simulink model "DoorLockCntr"  (R2019b)
settings: Solver=FixedStepDiscrete  StartTime=0.0  StopTime=10.0  FixedStep=0.1  RelTol=1e-3  EnableMultiTasking=on
undefined symbols (not defined in the file or in its folder): LockStatus, SpeedCntVal, SpeedTh
libraries: simulink x5
settings Model: DataDictionary=DoorLockCntr.sldd  EnableAccessToBaseWorkspace=off  Creator=yyamamot  LastModifiedBy=tliang
settings DataIOCC: LimitDataPoints=on  SaveOutput=off  SaveTime=off  ReturnWorkspaceOutputs=off
settings OptimizationCC: DefaultParameterBehavior=Inlined  UseFloatMulNetSlope=on  UseSpecifiedMinMax=on  InlineInvariantSignals=on  PassReuseOutputArgsAs=Individual arguments  ZeroExternalMemoryAtStartup=off  ZeroInternalMemoryAtStartup=off  NoFixptDivByZeroProtection=on  EfficientFloat2IntCast=on  LifeSpan=1  EfficientTunableParamExpr=on
settings DebuggingCC: SFUnexpectedBacktrackingDiag=warning  SFNoUnconditionalDefaultTransitionDiag=warning  SFExecutionAtInitializationDiag=none  ArithmeticOperatorsInVariantConditions=warning
settings HardwareCC: ProdBitPerPointer=32  ProdBitPerSizeT=32  ProdBitPerPtrDiffT=32  ProdLargestAtomicFloat=None  ProdWordSize=32  ProdHWDeviceType=Generic->32-bit Embedded Processor
settings ModelReferenceCC: ModelReferenceNumInstancesAllowed=Single  PropagateSignalLabelsOutOfModel=off
settings SFSimCC: SimUseLocalCustomCode=off  MATLABDynamicMemAlloc=off  CustomCodeUndefinedFunction=UseInterfaceOnly
settings RTWCC: SystemTargetFile=ert.tlc  TemplateMakefile=ert_default_tmf  GenerateReport=on  RTWVerbose=off  RTWUseLocalCustomCode=off  BuildConfiguration=Faster Runs  IncludeHyperlinkInReport=on  LaunchReport=on  PortableWordSizes=on  GenerateTraceInfo=on  GenerateTraceReport=on  GenerateTraceReportSl=on  GenerateTraceReportSf=on  GenerateTraceReportEml=on  GenerateWebview=on  GenerateCodeMetricsReport=on
settings CodeAppCC: IgnoreCustomStorageClasses=off  StateflowObjectComments=on  ReqsInCode=on
settings ERTTargetCC: UtilityFuncGeneration=Shared location  MultiwordLength=2048  GenerateSampleERTMain=on  IncludeMdlTerminateFcn=off  CombineSignalStateStructs=on  SuppressErrorStatus=on  SupportAbsoluteTime=off  SupportNonFinite=off  SupportComplex=off  ERTCustomFileTemplate=example_file_process.tlc  ERTFilePackagingFormat=Compact
settings ConfigComp: CovScope=ReferencedModels  CovIncludeTopModel=off  CovMetricSettings=dw  CovHtmlReporting=on  CovSaveCumulativeToWorkspaceVar=on  CovSaveSingleToWorkspaceVar=on  CovExternalEMLEnable=off  DVModelCoverageObjectives=MCDC  DVMaxTestCaseSteps=500  DVTestSuiteOptimization=LongTestcases

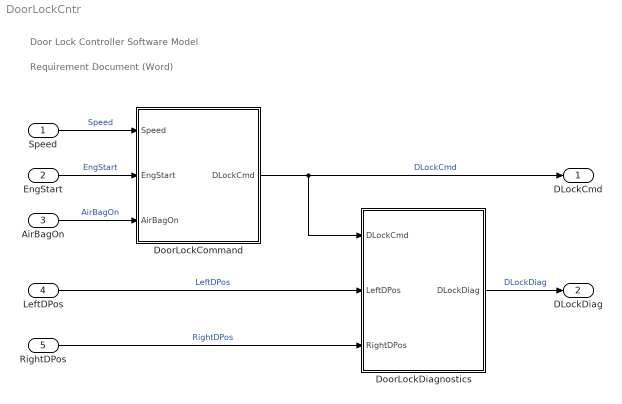
== system DoorLockCntr ==
  note: Door Lock Controller Software Model
  note: Requirement Document (Word)
  Speed : Inport  OutDataTypeStr=single  PortDimensions=1  SampleTime=0.1
  EngStart : Inport  Port=2  OutDataTypeStr=boolean  PortDimensions=1  SampleTime=0.1
  AirBagOn : Inport  Port=3  OutDataTypeStr=boolean  PortDimensions=1  SampleTime=0.1
  LeftDPos : Inport  Port=4  OutDataTypeStr=single  PortDimensions=1  SampleTime=0.1
  RightDPos : Inport  Port=5  OutDataTypeStr=single  PortDimensions=1  SampleTime=0.1
  DoorLockCommand : Subsystem  RequirementInfo={} %GIDa_0490e0d5_a34a_4647_aab7_4c3b06878525
  DoorLockDiagnostics : Subsystem  RequirementInfo={} %GIDa_5eeea999_d014_42a1_bdec_630b38744e2e
  DLockCmd : Outport  VectorParamsAs1DForOutWhenUnconnected=off
  DLockDiag : Outport  Port=2  VectorParamsAs1DForOutWhenUnconnected=off
  wires:
  DoorLockCommand/1(DLockCmd) -> DLockCmd/1, DoorLockDiagnostics/1(DLockCmd)  "DLockCmd"
  Speed/1 -> DoorLockCommand/1(Speed)  "Speed"
  EngStart/1 -> DoorLockCommand/2(EngStart)  "EngStart"
  AirBagOn/1 -> DoorLockCommand/3(AirBagOn)  "AirBagOn"
  LeftDPos/1 -> DoorLockDiagnostics/2(LeftDPos)  "LeftDPos"
  RightDPos/1 -> DoorLockDiagnostics/3(RightDPos)  "RightDPos"
  DoorLockDiagnostics/1(DLockDiag) -> DLockDiag/1  "DLockDiag"

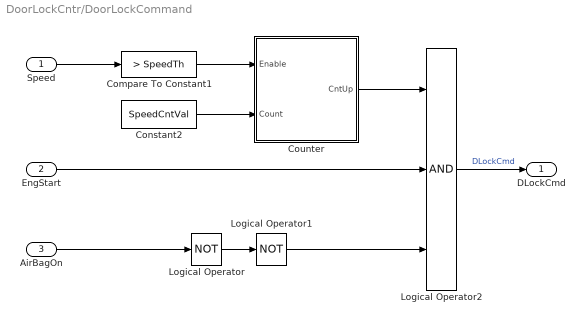
== system DoorLockCntr/DoorLockCommand ==
  Speed : Inport
  EngStart : Inport  Port=2
  AirBagOn : Inport  Port=3
  Compare To Constant1 : simulink/Logic and Bit Operations/Compare To Constant  relop=>  const=SpeedTh  OutDataTypeStr=boolean
  Constant2 : Constant  Value=SpeedCntVal  OutDataTypeStr=uint8
      settings: AttributesFormatString=DataType = %<OutDataTypeStr>
  Counter : Subsystem
  Logical Operator : Logic  Operator=NOT  AllPortsSameDT=off  OutDataTypeStr=boolean
  Logical Operator1 : Logic  Operator=NOT  AllPortsSameDT=off  OutDataTypeStr=boolean
  Logical Operator2 : Logic  Inputs=3  AllPortsSameDT=off  OutDataTypeStr=boolean
  DLockCmd : Outport  VectorParamsAs1DForOutWhenUnconnected=off
  wires:
  Speed/1 -> Compare To Constant1/1
  Logical Operator2/1 -> DLockCmd/1  "DLockCmd"
  Compare To Constant1/1 -> Counter/1(Enable)
  Constant2/1 -> Counter/2(Count)
  Counter/1(CntUp) -> Logical Operator2/1
  EngStart/1 -> Logical Operator2/2
  AirBagOn/1 -> Logical Operator/1
  Logical Operator/1 -> Logical Operator1/1
  Logical Operator1/1 -> Logical Operator2/3

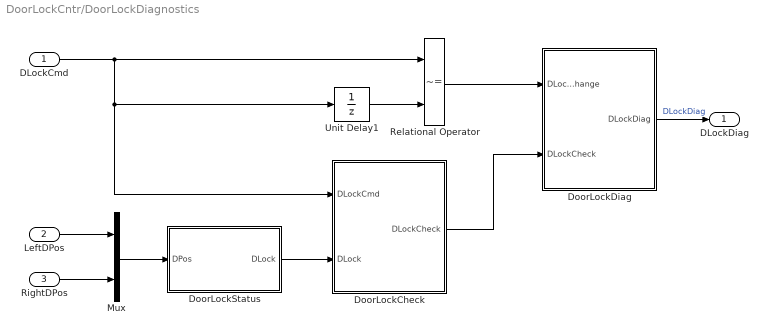
== system DoorLockCntr/DoorLockDiagnostics ==
  DLockCmd : Inport
  LeftDPos : Inport  Port=2
  RightDPos : Inport  Port=3
  DoorLockCheck : Subsystem
  DoorLockDiag : Stateflow chart  TreatAsAtomicUnit=on
  DoorLockStatus : Subsystem
  Mux : Mux  Inputs=2
  Relational Operator : RelationalOperator  Operator=~=  OutDataTypeStr=boolean  RndMeth=Nearest
  Unit Delay1 : UnitDelay  SampleTime=-1  StateName=DLockCmd_prev  HasFrameUpgradeWarning=on  StateMustResolveToSignalObject=on
      settings: AttributesFormatString=InitialValue = %<InitialCondition>\nState = %<StateName>
  DLockDiag : Outport  VectorParamsAs1DForOutWhenUnconnected=off
  wires:
  DoorLockStatus/1(DLock) -> DoorLockCheck/2(DLock)
  Mux/1 -> DoorLockStatus/1(DPos)
  LeftDPos/1 -> Mux/1
  RightDPos/1 -> Mux/2
  DoorLockCheck/1(DLockCheck) -> DoorLockDiag/2(DLockCheck)
  DoorLockDiag/1(DLockDiag) -> DLockDiag/1  "DLockDiag"
  DLockCmd/1 -> DoorLockCheck/1(DLockCmd), Unit Delay1/1, Relational Operator/1
  Unit Delay1/1 -> Relational Operator/2
  Relational Operator/1 -> DoorLockDiag/1(DLockCmdChange)

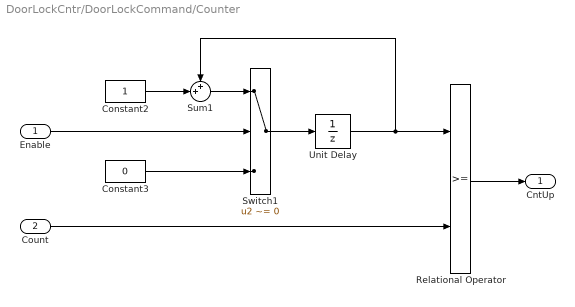
== system DoorLockCntr/DoorLockCommand/Counter ==
  Enable : Inport
  Count : Inport  Port=2
  Constant2 : Constant  OutDataTypeStr=uint8
      settings: AttributesFormatString=DataType = %<OutDataTypeStr>
  Constant3 : Constant  Value=0  OutDataTypeStr=uint8
      settings: AttributesFormatString=DataType = %<OutDataTypeStr>
  Relational Operator : RelationalOperator  OutDataTypeStr=boolean  RndMeth=Nearest
  Sum1 : Sum  Inputs=++|  RndMeth=Simplest  SaturateOnIntegerOverflow=on
      settings: AttributesFormatString=SatInt = %<SaturateOnIntegerOverflow>
  Switch1 : Switch  Criteria=u2 ~= 0  RndMeth=Simplest
  Unit Delay : UnitDelay  SampleTime=-1  StateName=SpeedCnt  HasFrameUpgradeWarning=on  StateMustResolveToSignalObject=on
      settings: AttributesFormatString=InitialValue = %<InitialCondition>\nState = %<StateName>
  CntUp : Outport  VectorParamsAs1DForOutWhenUnconnected=off
  wires:
  Enable/1 -> Switch1/2
  Constant3/1 -> Switch1/3
  Switch1/1 -> Unit Delay/1
  Unit Delay/1 -> Relational Operator/1, Sum1/1
  Sum1/1 -> Switch1/1
  Constant2/1 -> Sum1/2
  Count/1 -> Relational Operator/2
  Relational Operator/1 -> CntUp/1

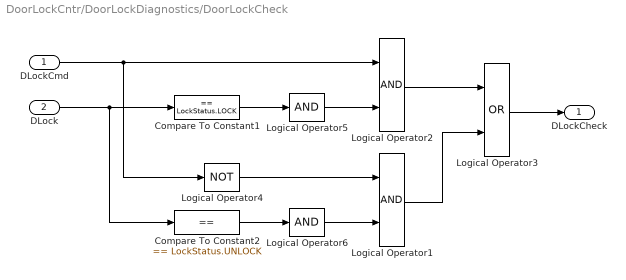
== system DoorLockCntr/DoorLockDiagnostics/DoorLockCheck ==
  DLockCmd : Inport
  DLock : Inport  Port=2
  Compare To Constant1 : simulink/Logic and Bit Operations/Compare To Constant  relop===  const=LockStatus.LOCK  OutDataTypeStr=boolean
  Compare To Constant2 : simulink/Logic and Bit Operations/Compare To Constant  relop===  const=LockStatus.UNLOCK  OutDataTypeStr=boolean
  Logical Operator1 : Logic  AllPortsSameDT=off  OutDataTypeStr=boolean
  Logical Operator2 : Logic  AllPortsSameDT=off  OutDataTypeStr=boolean
  Logical Operator3 : Logic  Operator=OR  AllPortsSameDT=off  OutDataTypeStr=boolean
  Logical Operator4 : Logic  Operator=NOT  AllPortsSameDT=off  OutDataTypeStr=boolean
  Logical Operator5 : Logic  Inputs=1  AllPortsSameDT=off  OutDataTypeStr=boolean
  Logical Operator6 : Logic  Inputs=1  AllPortsSameDT=off  OutDataTypeStr=boolean
  DLockCheck : Outport  VectorParamsAs1DForOutWhenUnconnected=off
  wires:
  Logical Operator3/1 -> DLockCheck/1
  DLock/1 -> Compare To Constant1/1, Compare To Constant2/1
  Compare To Constant1/1 -> Logical Operator5/1
  DLockCmd/1 -> Logical Operator4/1, Logical Operator2/1
  Logical Operator4/1 -> Logical Operator1/1
  Compare To Constant2/1 -> Logical Operator6/1
  Logical Operator2/1 -> Logical Operator3/1
  Logical Operator1/1 -> Logical Operator3/2
  Logical Operator5/1 -> Logical Operator2/2
  Logical Operator6/1 -> Logical Operator1/2

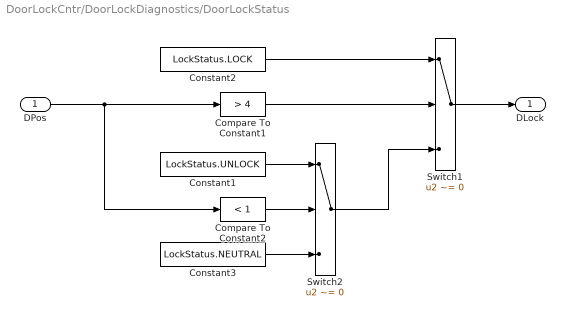
== system DoorLockCntr/DoorLockDiagnostics/DoorLockStatus ==
  DPos : Inport
  Compare To Constant1 : simulink/Logic and Bit Operations/Compare To Constant  relop=>  const=4  OutDataTypeStr=boolean
  Compare To Constant2 : simulink/Logic and Bit Operations/Compare To Constant  relop=<  const=1  OutDataTypeStr=boolean
  Constant1 : Constant  Value=LockStatus.UNLOCK  OutDataTypeStr=Enum: LockStatus
      settings: AttributesFormatString=DataType = %<OutDataTypeStr>
  Constant2 : Constant  Value=LockStatus.LOCK  OutDataTypeStr=Enum: LockStatus
      settings: AttributesFormatString=DataType = %<OutDataTypeStr>
  Constant3 : Constant  Value=LockStatus.NEUTRAL  OutDataTypeStr=Enum: LockStatus
      settings: AttributesFormatString=DataType = %<OutDataTypeStr>
  Switch1 : Switch  Criteria=u2 ~= 0  RndMeth=Simplest
  Switch2 : Switch  Criteria=u2 ~= 0  RndMeth=Simplest
  DLock : Outport  VectorParamsAs1DForOutWhenUnconnected=off
  wires:
  Compare To Constant1/1 -> Switch1/2
  Constant2/1 -> Switch1/1
  Switch2/1 -> Switch1/3
  Compare To Constant2/1 -> Switch2/2
  Constant1/1 -> Switch2/1
  Constant3/1 -> Switch2/3
  DPos/1 -> Compare To Constant1/1, Compare To Constant2/1
  Switch1/1 -> DLock/1

== stateflow chart DoorLockCntr/DoorLockDiagnostics/DoorLockDiag ==
  state NORMAL
    entry:
    DLockDiag = NORMAL;
  state WARNING
    entry:
    DiagCnt = 1;
    during:
    DiagCnt++;
  state FAIL
    entry:
    DLockDiag = FAIL;
  (default) -> NORMAL
  NORMAL -> WARNING : [DLockCmdChange]
  (junction 7) -> NORMAL [order 1] : [DLockCheck]
  WARNING -> WARNING [order 1] : [!DLockCmdChange]
  WARNING -> (junction 7) [order 2] : [DiagCnt == DiagCntVal]
  (junction 7) -> FAIL [order 2]
  data: DLockCmdChange input; DLockCheck input; DLockDiag output Enum: DiagStatus; DiagCnt local uint8; DiagCntVal parameter
